simulink model "Symulacja_dobor_regulatora"  (R2022b)
settings: Solver=VariableStepAuto  StartTime=0.0  StopTime=1000.0  RelTol=1e-3
libraries: slpidlib x1
settings Model: Creator=User  LastModifiedBy=User

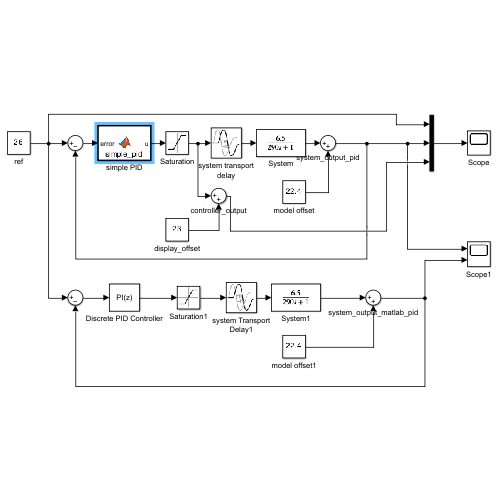
[thumbnail: Simulink's stored preview of the top-level diagram]
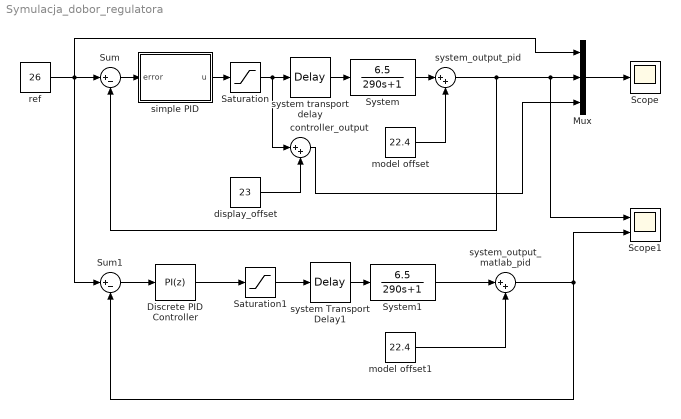
== system Symulacja_dobor_regulatora ==
  Discrete PID Controller : slpidlib/PID Controller  Controller=PI  Form=Parallel  TimeDomain=Discrete-time  UseExternalTs=off  SampleTime=1  IntegratorMethod=Trapezoidal  FilterMethod=Backward Euler  ControllerParametersSource=internal  P=1.54872967509146  I=0.0184338237431332  UseKiTs=off  D=4.42552163053413  N=0.0108550498735103  UseFilter=on  TunerSelectOption=Transfer Function Based (PID Tuner App)  InitialConditionSource=internal  InitialConditionForIntegrator=0  InitialConditionForFilter=0  DifferentiatorICPrevScaledInput=0  ExternalReset=none  TrackingMode=off  Kt=1  LimitOutput=off  SatLimitsSource=internal  UpperSaturationLimit=inf  LowerSaturationLimit=-inf  LinearizeAsGain=off  AntiWindupMode=none  Kb=1  LimitIntegrator=off  UpperIntegratorSaturationLimit=inf  LowerIntegratorSaturationLimit=-inf  POutMin=[]  POutMax=[]  IOutMin=[]  IOutMax=[]  DOutMin=[]  DOutMax=[]  NOutMin=[]  NOutMax=[]  SumOutMin=[]  SumOutMax=[]  SaturationOutMin=[]  SaturationOutMax=[]  PParamMin=[]  PParamMax=[]  IParamMin=[]  IParamMax=[]  DParamMin=[]  DParamMax=[]  NParamMin=[]  NParamMax=[]  KbParamMin=[]  KbParamMax=[]  KtParamMin=[]  KtParamMax=[]  KbOutMin=[]  KbOutMax=[]  KtOutMin=[]  KtOutMax=[]  IntegratorOutMin=[]  IntegratorOutMax=[]  FilterOutMin=[]  FilterOutMax=[]  SumI1OutMin=[]  SumI1OutMax=[]  SumI2OutMin=[]  SumI2OutMax=[]  SumI3OutMin=[]  SumI3OutMax=[]  SumI4OutMin=[]  SumI4OutMax=[]  SumDOutMin=[]  SumDOutMax=[]  DifferentiatorOutMin=[]  DifferentiatorOutMax=[]  FilterDiffOutCoefMin=[]  FilterDiffOutCoefMax=[]  ReciprocalOutMin=[]  ReciprocalOutMax=[]  SumDenOutMin=[]  SumDenOutMax=[]  SumNumOutMin=[]  SumNumOutMax=[]  DivideOutMin=[]  DivideOutMax=[]  UdiffTsProdOutMin=[]  UdiffTsProdOutMax=[]  NTsProdOutMin=[]  NTsProdOutMax=[]  UintegralTsProdOutMin=[]  UintegralTsProdOutMax=[]  UngainTsProdOutMin=[]  UngainTsProdOutMax=[]  ClampingZeroOutDataTypeStr=Inherit: Inherit via back propagation  ClampingZeroOutMin=[]  ClampingZeroOutMax=[]  FilterDenConstantOutDataTypeStr=Inherit: Inherit via back propagation  FilterDenConstantOutMin=[]  FilterDenConstantOutMax=[]  PCopyOutDataTypeStr=Inherit: Inherit via back propagation  PCopyOutMin=[]  PCopyOutMax=[]  NCopyOutDataTypeStr=Inherit: Inherit via back propagation  NCopyOutMin=[]  NCopyOutMax=[]  IntegratorContinuousStateAttributes=''  IntegratorStateMustResolveToSignalObject=off  IntegratorRTWStateStorageClass=Auto  FilterContinuousStateAttributes=''  FilterStateMustResolveToSignalObject=off  FilterRTWStateStorageClass=Auto  ParallelPVariant=InternalParameters  IdealPVariant=Disabled  IVariant=InternalParameters  DVariant=Disabled  IntegratorVariant=Discrete  SatVariant=Disabled  AWVariant=Passthrough  PCopyVariant=Disabled  TRVariant=Disabled  FdbkBlocksVariant=Forward  IdealPFdbkVariant=Disabled  SatFdbkVariant=Disabled  DerivativeFilterVariant=Disabled  NVariant=Disabled  NCopyVariant=Disabled_SignalSpec  FilterICVariant=Disabled  IntegratorICVariant=InternalICs  ExternalResetVariant=Disabled  TRSumVariant=Passthrough  SumFdbkVariant=Disabled  SumVariant=Sum_PI  TsampFilterVariant=InternalTs  TsampNgainVariant=Passthrough  TsampIntegralVariant=Passthrough  ExternalSaturationOutDataTypeStr=Inherit: Same as second input
      settings: LibrarySourceBlock=simulink/Discrete/Discrete PID Controller
  Mux : Mux  Inputs=3
  Saturation : Saturate  UpperLimit=1  LowerLimit=0
  Saturation1 : Saturate  UpperLimit=1  LowerLimit=0
  Scope : Scope
  Scope1 : Scope  NumInputPorts=2
  Sum : Sum  Inputs=|+-
  Sum1 : Sum  Inputs=|+-
  System : TransferFcn  Numerator=[6.5]  Denominator=[290 1]
  System1 : TransferFcn  Numerator=[6.5]  Denominator=[290 1]
  controller_output : Sum  Inputs=|++
  display_offset : Constant  Value=23
  model offset : Constant  Value=22.4
  model offset1 : Constant  Value=22.4
  ref : Constant  Value=26
  simple PID : MATLAB Function  TreatAsAtomicUnit=on
  system Transport Delay1 : TransportDelay  DelayTime=15
  system transport delay : TransportDelay  DelayTime=15
  system_output_matlab_pid : Sum  Inputs=|++
  system_output_pid : Sum  Inputs=|++
  wires:
  Sum/1 -> simple PID/1(error)
  simple PID/1(u) -> Saturation/1
  Saturation/1 -> controller_output/1, system transport delay/1
  display_offset/1 -> controller_output/2
  system transport delay/1 -> System/1
  System/1 -> system_output_pid/1
  model offset/1 -> system_output_pid/2
  Mux/1 -> Scope/1
  system_output_pid/1 -> Sum/2, Mux/2, Scope1/1
  ref/1 -> Sum/1, Mux/1, Sum1/1
  controller_output/1 -> Mux/3
  system_output_matlab_pid/1 -> Scope1/2, Sum1/2
  Sum1/1 -> Discrete PID Controller/1
  Discrete PID Controller/1 -> Saturation1/1
  Saturation1/1 -> system Transport Delay1/1
  system Transport Delay1/1 -> System1/1
  System1/1 -> system_output_matlab_pid/1
  model offset1/1 -> system_output_matlab_pid/2

== matlab function Symulacja_dobor_regulatora/simple PID ==
  settings: updateMethod=DISCRETE  sampleTime=1
  data: error input; u output
function u = simple_pid(error)

%Declare static value
persistent previous_error;
if isempty (previous_error)
    previous_error = 0;
end

persistent previous_integral;
if isempty (previous_integral)
    previous_integral = 0;
end

%Constant values
dt = 1;
Kp = 1.54872967509146;
Ki = 0.0184338237431332;
Kd = 0;
N = 100;

%proportional part
P = Kp*error;

%integral part
integral = previous_integral + (error + previous_error); %numerical integrator without anti-windup
previous_integral = integral;
I = Ki*integral*(dt/2);

%derivative part
derivative = (error - previous_error)/dt; %numerical derivative without filter
previous_error = error;
D = Kd*derivative;


%sum of all parts
u = P + I + D; %without saturation
